simulink model "JenaFox_Klostermair_Neuronal_Controller"  (R2020b)
settings: Solver=ode23s  StartTime=0.0  StopTime=20  MaxStep=maxStep  RelTol=relTol  AbsTol=absTol
InitFcn:
  | Fox_param;
undefined symbols (not defined in the file or in its folder): amplifier, c_coupling_hip, c_coupling_knee, c_hs, d_coupling_knee, d_hs, g, hip_i, hip_Jm, hip_k, hip_Mrg, hip_Mrhg, hip_na, hip_Ra, IC_motor_hip_l, IC_motor_hip_r, IC_motor_knee_l, IC_motor_knee_r, IC_phi_hip_l, IC_phi_hip_r, IC_v_motor_hip, IC_v_motor_knee, k_gx, k_gy, knee_i, knee_Jm, knee_k, knee_Mrg, knee_Mrhg, knee_na, knee_Ra, mu_slide, mu_stick, smiData, v_gx_max, v_gy_max, vLimit, X, Y, Z
libraries: sm_lib x38, nesl_utility x26, simulink x16, simulink_extras x8
(part 2 of 3)

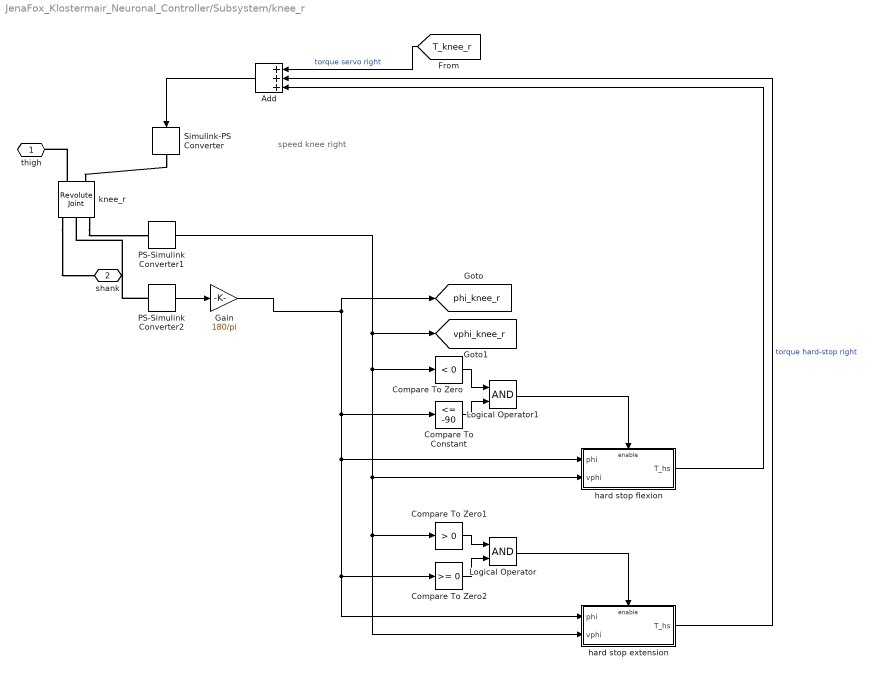
== system JenaFox_Klostermair_Neuronal_Controller/Subsystem/knee_r ==
  note: speed knee right
  Add : Sum  Inputs=+++
  Compare To Constant : simulink/Logic and Bit Operations/Compare To Constant  relop=<=  const=-90  OutDataTypeStr=uint8
  Compare To Zero : simulink/Logic and Bit Operations/Compare To Zero  relop=<  OutDataTypeStr=uint8  ZeroCross=off
  Compare To Zero1 : simulink/Logic and Bit Operations/Compare To Zero  relop=>  OutDataTypeStr=uint8  ZeroCross=off
  Compare To Zero2 : simulink/Logic and Bit Operations/Compare To Zero  relop=>=  OutDataTypeStr=uint8
  Gain : Gain  Gain=180/pi
  Logical Operator : Logic  AllPortsSameDT=off  OutDataTypeStr=boolean
  Logical Operator1 : Logic  AllPortsSameDT=off  OutDataTypeStr=boolean
  PS-Simulink Converter1 : nesl_utility/PS-Simulink Converter  PhysicalDomain=network_engine_domain  SubClassName=ps_output  LeftPortType=input  RightPortType=output  PseudoPeriodic=off  Frequencies=[]  Unit=1  AffineConversion=off
  PS-Simulink Converter2 : nesl_utility/PS-Simulink Converter  PhysicalDomain=network_engine_domain  SubClassName=ps_output  LeftPortType=input  RightPortType=output  PseudoPeriodic=off  Frequencies=[]  Unit=1  AffineConversion=off
  Simulink-PS Converter : nesl_utility/Simulink-PS Converter  PhysicalDomain=network_engine_domain  SubClassName=ps_input  LeftPortType=input  RightPortType=output  PseudoPeriodic=off  Frequencies=[]  NoiseDistribution=none  NoiseParameters=[]  Unit=1  AffineConversion=off  FilteringAndDerivatives=provide  SimscapeFilterOrder=1  InputFilterTimeConstant=0.001  UdotUserProvided=0
  hard stop extension : Subsystem  TreatAsAtomicUnit=on
  hard stop flexion : Subsystem  TreatAsAtomicUnit=on
  knee_r : sm_lib/Joints/Revolute Joint  JointMode=Normal  SenseConstraintForce=off  SenseConstraintForceX=off  SenseConstraintForceY=off  SenseConstraintForceZ=off  SenseConstraintTorque=off  SenseConstraintTorqueX=off  SenseConstraintTorqueY=off  SenseConstraintTorqueZ=off  SenseTotalForce=off  SenseTotalForceX=off  SenseTotalForceY=off  SenseTotalForceZ=off  SenseTotalTorque=off  SenseTotalTorqueX=off  SenseTotalTorqueY=off  SenseTotalTorqueZ=off  CompositeWrenchDir=FollowerOnBase  CompositeWrenchFrame=BaseFrame  EquilibriumPosition=0  EquilibriumPositionUnits=rad  SpringStiffness=0  SpringStiffnessUnits=N*m/rad  DampingCoefficient=d_joint  DampingCoefficientUnits=N*m/(rad/s)  TorqueActuationMode=InputTorque  MotionActuationMode=ComputedMotion  SensePosition=on  SenseVelocity=on  SenseAcceleration=off  SenseTorqueForce=off  SenseLowerLimitTorqueForce=off  SenseUpperLimitTorqueForce=off  LowerLimitSpecify=off  LowerLimitBound=-90  LowerLimitBoundUnits=deg  LowerLimitStiffness=1e4  LowerLimitStiffnessUnits=N*m/deg  LowerLimitDamping=10  LowerLimitDampingUnits=N*m/(deg/s)  LowerLimitTransitionRegionWidth=0.1  LowerLimitTransitionRegionWidthUnits=deg  UpperLimitSpecify=off  UpperLimitBound=90  UpperLimitBoundUnits=deg  UpperLimitStiffness=1e4  UpperLimitStiffnessUnits=N*m/deg  UpperLimitDamping=10  UpperLimitDampingUnits=N*m/(deg/s)  UpperLimitTransitionRegionWidth=0.1  UpperLimitTransitionRegionWidthUnits=deg  PositionTargetSpecify=on  PositionTargetPriority=High  PositionTargetValue=IC_phi_knee_r  PositionTargetValueUnits=deg  VelocityTargetSpecify=off  VelocityTargetPriority=High  VelocityTargetValue=0  VelocityTargetValueUnits=deg/s
  thigh : PMIOPort  Side=Left
  shank : PMIOPort  Port=2  Side=Right
  tag scope: phi_knee_r=global, vphi_knee_r=global
  wires:
  Compare To Constant/1 -> Logical Operator1/2
  PS-Simulink Converter2/1 -> Gain/1
  hard stop extension/1(T_hs) -> Add/2  "torque hard-stop right"
  Compare To Zero1/1 -> Logical Operator/1
  Logical Operator1/1 -> hard stop flexion/Enable
  Logical Operator/1 -> hard stop extension/Enable
  Add/1 -> Simulink-PS Converter/1
  Compare To Zero/1 -> Logical Operator1/1
  PS-Simulink Converter1/1 -> [vphi_knee_r], Compare To Zero/1, hard stop flexion/2(vphi), Compare To Zero1/1, hard stop extension/2(vphi)
  hard stop flexion/1(T_hs) -> Add/3
  Compare To Zero2/1 -> Logical Operator/2
  [T_knee_r] -> Add/1  "torque servo right"
  Gain/1 -> [phi_knee_r], Compare To Constant/1, hard stop flexion/1(phi), Compare To Zero2/1, hard stop extension/1(phi)
  connections:
  Simulink-PS Converter/RConn1 -- knee_r/LConn2
  knee_r/RConn1 -- shank/RConn1
  PS-Simulink Converter2/LConn1 -- knee_r/RConn2
  knee_r/RConn3 -- PS-Simulink Converter1/LConn1
  knee_r/LConn1 -- thigh/RConn1

== system JenaFox_Klostermair_Neuronal_Controller/Subsystem/shank_bottom_l ==
  Rigid Transform : sm_lib/Frames and Transforms/Rigid Transform  TranslationMethod=None  TranslationStandardOffset=0  TranslationLengthUnit=m  TranslationStandardAxis=+Z  TranslationCartesianOffset=[0 0 0]  TranslationROffset=0  TranslationROffsetUnits=m  TranslationZOffset=0  TranslationZOffsetUnits=m  TranslationThetaOffset=0  TranslationThetaOffsetUnits=deg  RotationMethod=AlignedAxes  RotationAngleUnits=deg  RotationStandardAxis=+Z  RotationAngle=0.0  RotationArbitraryAxis=[0 0 1]  FollAlignAxisA=+X  BaseAlignAxisA=-X  FollAlignAxisB=+Z  BaseAlignAxisB=+Y  RotationSequenceAxes=FollowerAxes  RotationSequence=XYX  RotationSequenceAngles=[0 0 0]  RotationSequenceAnglesUnits=deg  RotationMatrix=[1 0 0; 0 1 0; 0 0 1]
  Solid : sm_lib/Body Elements/File Solid  ExtGeomFileName=shank_bottom_ipt_92530788.STEP  UnitType=FromFile  ExtGeomFileUnits=m  StepReaderType=OCC  ExportConvexHullGeometry=off  InertiaType=Custom  Mass=smiData.Solid(4).mass  MassUnits=kg  CenterOfMass=smiData.Solid(4).CoM  CenterOfMassUnits=mm  MomentsOfInertia=smiData.Solid(4).MoI  MomentsOfInertiaUnits=kg*mm^2  ProductsOfInertia=smiData.Solid(4).PoI  ProductsOfInertiaUnits=kg*mm^2  BasedOnType=Density  Density=1000  DensityUnits=kg/m^3  DoExposeReferenceFrame=on  SerializedFrames=<Frames><Frame><Id>Frame1</Id><Value><Name>ground_contact</Name><Origin><Source>GeometricFeature</Source><FeatureName>circular curve 105</FeatureName></Origin><PrimaryAxis><DefinedDirection>+Y</DefinedDirection><Source>ReferenceFrame</Source><SourceDirection>-Y</SourceDirection><FeatureName></FeatureName></PrimaryAxis><SecondaryAxis><DefinedDirection>+X</DefinedDirection><Source>ReferenceFrame</Source><SourceDirection>+X</SourceDirection><FeatureName></FeatureName></SecondaryAxis></Value></Frame><Frame><Id>Frame2</Id><Value><Name>spring_bottom</Name><Origin><Source>GeometricFeature</Source><FeatureName>circular curve 81</FeatureName></Origin><PrimaryAxis><DefinedDirection>+Y</DefinedDirection><Source>ReferenceFrame</Source><SourceDirection>-Y</SourceDirection><FeatureName></FeatureName></PrimaryAxis><SecondaryAxis><DefinedDirection>+X</DefinedDirection><Source>ReferenceFrame</Source><SourceDirection>+X</SourceDirection><FeatureName></FeatureName></SecondaryAxis></Value></Frame></Frames>  GraphicType=FromGeometry  MarkerShape=Sphere  MarkerSize=10  GraphicVisPropType=SimpleVisualProperties  GraphicDiffuseColor=smiData.Solid(4).color  GraphicSpecularColor=[0.5 0.5 0.5 1.0]  GraphicAmbientColor=[0.15 0.15 0.15 1.0]  GraphicEmissiveColor=[0.0 0.0 0.0 1.0]  GraphicShininess=75  GraphicOpacity=smiData.Solid(4).opacity
  linear elastic joint : PMIOPort  Side=Left
  toe : PMIOPort  Port=2  Side=Right
  spring_bottom : PMIOPort  Port=3  Side=Left
  connections:
  toe/RConn1 -- Solid/LConn1
  linear elastic joint/RConn1 -- Rigid Transform/RConn1 -- spring_bottom/RConn1
  Rigid Transform/LConn1 -- Solid/LConn2

== system JenaFox_Klostermair_Neuronal_Controller/Subsystem/shank_bottom_r ==
  Rigid Transform : sm_lib/Frames and Transforms/Rigid Transform  TranslationMethod=None  TranslationStandardOffset=0  TranslationLengthUnit=m  TranslationStandardAxis=+Z  TranslationCartesianOffset=[0 0 0]  TranslationROffset=0  TranslationROffsetUnits=m  TranslationZOffset=0  TranslationZOffsetUnits=m  TranslationThetaOffset=0  TranslationThetaOffsetUnits=deg  RotationMethod=AlignedAxes  RotationAngleUnits=deg  RotationStandardAxis=+Z  RotationAngle=0.0  RotationArbitraryAxis=[0 0 1]  FollAlignAxisA=+X  BaseAlignAxisA=+X  FollAlignAxisB=+Z  BaseAlignAxisB=+Y  RotationSequenceAxes=FollowerAxes  RotationSequence=XYX  RotationSequenceAngles=[0 0 0]  RotationSequenceAnglesUnits=deg  RotationMatrix=[1 0 0; 0 1 0; 0 0 1]
  Solid : sm_lib/Body Elements/File Solid  ExtGeomFileName=shank_bottom_ipt_92530788.STEP  UnitType=FromFile  ExtGeomFileUnits=m  StepReaderType=OCC  ExportConvexHullGeometry=off  InertiaType=Custom  Mass=smiData.Solid(4).mass  MassUnits=kg  CenterOfMass=smiData.Solid(4).CoM  CenterOfMassUnits=mm  MomentsOfInertia=smiData.Solid(4).MoI  MomentsOfInertiaUnits=kg*mm^2  ProductsOfInertia=smiData.Solid(4).PoI  ProductsOfInertiaUnits=kg*mm^2  BasedOnType=Density  Density=1000  DensityUnits=kg/m^3  DoExposeReferenceFrame=off  SerializedFrames=<Frames><Frame><Id>Frame1</Id><Value><Name>ground_contact</Name><Origin><Source>GeometricFeature</Source><FeatureName>circular curve 105</FeatureName></Origin><PrimaryAxis><DefinedDirection>+Y</DefinedDirection><Source>ReferenceFrame</Source><SourceDirection>-Y</SourceDirection><FeatureName></FeatureName></PrimaryAxis><SecondaryAxis><DefinedDirection>+X</DefinedDirection><Source>ReferenceFrame</Source><SourceDirection>+X</SourceDirection><FeatureName></FeatureName></SecondaryAxis></Value></Frame><Frame><Id>Frame2</Id><Value><Name>spring_bottom</Name><Origin><Source>GeometricFeature</Source><FeatureName>circular curve 81</FeatureName></Origin><PrimaryAxis><DefinedDirection>+Y</DefinedDirection><Source>ReferenceFrame</Source><SourceDirection>-Y</SourceDirection><FeatureName></FeatureName></PrimaryAxis><SecondaryAxis><DefinedDirection>+X</DefinedDirection><Source>ReferenceFrame</Source><SourceDirection>+X</SourceDirection><FeatureName></FeatureName></SecondaryAxis></Value></Frame></Frames>  GraphicType=FromGeometry  MarkerShape=Sphere  MarkerSize=10  GraphicVisPropType=SimpleVisualProperties  GraphicDiffuseColor=smiData.Solid(4).color  GraphicSpecularColor=[0.5 0.5 0.5 1.0]  GraphicAmbientColor=[0.15 0.15 0.15 1.0]  GraphicEmissiveColor=[0.0 0.0 0.0 1.0]  GraphicShininess=75  GraphicOpacity=smiData.Solid(4).opacity
  linear elastic joint : PMIOPort  Side=Left
  toe : PMIOPort  Port=2  Side=Right
  spring_bottom : PMIOPort  Port=3  Side=Left
  connections:
  toe/RConn1 -- Solid/LConn1
  linear elastic joint/RConn1 -- Rigid Transform/RConn1 -- spring_bottom/RConn1
  Rigid Transform/LConn1 -- Solid/RConn1

== system JenaFox_Klostermair_Neuronal_Controller/Subsystem/shank_top_l ==
  Rigid Transform : sm_lib/Frames and Transforms/Rigid Transform  TranslationMethod=StandardAxis  TranslationStandardOffset=0.11  TranslationLengthUnit=m  TranslationStandardAxis=+Z  TranslationCartesianOffset=[0 0 0]  TranslationROffset=0  TranslationROffsetUnits=m  TranslationZOffset=0  TranslationZOffsetUnits=m  TranslationThetaOffset=0  TranslationThetaOffsetUnits=deg  RotationMethod=AlignedAxes  RotationAngleUnits=deg  RotationStandardAxis=+Z  RotationAngle=0.0  RotationArbitraryAxis=[0 0 1]  FollAlignAxisA=+X  BaseAlignAxisA=+X  FollAlignAxisB=+Y  BaseAlignAxisB=+Z  RotationSequenceAxes=FollowerAxes  RotationSequence=XYX  RotationSequenceAngles=[0 0 0]  RotationSequenceAnglesUnits=deg  RotationMatrix=[1 0 0; 0 1 0; 0 0 1]
  Solid : sm_lib/Body Elements/File Solid  ExtGeomFileName=shank_top_ipt_5be12039.STEP  UnitType=FromFile  ExtGeomFileUnits=m  StepReaderType=OCC  ExportConvexHullGeometry=off  InertiaType=Custom  Mass=smiData.Solid(3).mass  MassUnits=kg  CenterOfMass=smiData.Solid(3).CoM  CenterOfMassUnits=mm  MomentsOfInertia=smiData.Solid(3).MoI  MomentsOfInertiaUnits=kg*mm^2  ProductsOfInertia=smiData.Solid(3).PoI  ProductsOfInertiaUnits=kg*mm^2  BasedOnType=Density  Density=1000  DensityUnits=kg/m^3  DoExposeReferenceFrame=off  SerializedFrames=<Frames><Frame><Id>Frame1</Id><Value><Name>spring_top</Name><Origin><Source>GeometricFeature</Source><FeatureName>circular curve 166</FeatureName></Origin><PrimaryAxis><DefinedDirection>+Y</DefinedDirection><Source>ReferenceFrame</Source><SourceDirection>-Y</SourceDirection><FeatureName></FeatureName></PrimaryAxis><SecondaryAxis><DefinedDirection>+X</DefinedDirection><Source>GeometricFeature</Source><SourceDirection>+X</SourceDirection><FeatureName>segment 110</FeatureName></SecondaryAxis></Value></Frame><Frame><Id>Frame2</Id><Value><Name>knee</Name><Origin><Source>GeometricFeature</Source><FeatureName>circular curve 135</FeatureName></Origin><PrimaryAxis><DefinedDirection>-X</DefinedDirection><Source>GeometricFeature</Source><SourceDirection>+Z</SourceDirection><FeatureName>segment 80</FeatureName></PrimaryAxis><SecondaryAxis><DefinedDirection>+Y</DefinedDirection><Source>GeometricFeature</Source><SourceDirection>+X</SourceDirection><FeatureName>segment 115</FeatureName></SecondaryAxis></Value></Frame></Frames>  GraphicType=FromGeometry  MarkerShape=Sphere  MarkerSize=10  GraphicVisPropType=SimpleVisualProperties  GraphicDiffuseColor=smiData.Solid(3).color  GraphicSpecularColor=[0.5 0.5 0.5 1.0]  GraphicAmbientColor=[0.15 0.15 0.15 1.0]  GraphicEmissiveColor=[0.0 0.0 0.0 1.0]  GraphicShininess=75  GraphicOpacity=smiData.Solid(3).opacity
  knee : PMIOPort  Side=Left
  linear joint : PMIOPort  Port=2  Side=Right
  spring_top : PMIOPort  Port=3  Side=Right
  connections:
  knee/RConn1 -- Solid/RConn1
  Rigid Transform/RConn1 -- spring_top/RConn1 -- Solid/LConn1
  linear joint/RConn1 -- Rigid Transform/LConn1

== system JenaFox_Klostermair_Neuronal_Controller/Subsystem/shank_top_r ==
  Rigid Transform : sm_lib/Frames and Transforms/Rigid Transform  TranslationMethod=StandardAxis  TranslationStandardOffset=0.11  TranslationLengthUnit=m  TranslationStandardAxis=+Z  TranslationCartesianOffset=[0 0 0]  TranslationROffset=0  TranslationROffsetUnits=m  TranslationZOffset=0  TranslationZOffsetUnits=m  TranslationThetaOffset=0  TranslationThetaOffsetUnits=deg  RotationMethod=AlignedAxes  RotationAngleUnits=deg  RotationStandardAxis=+Z  RotationAngle=0.0  RotationArbitraryAxis=[0 0 1]  FollAlignAxisA=+X  BaseAlignAxisA=+X  FollAlignAxisB=+Y  BaseAlignAxisB=+Z  RotationSequenceAxes=FollowerAxes  RotationSequence=XYX  RotationSequenceAngles=[0 0 0]  RotationSequenceAnglesUnits=deg  RotationMatrix=[1 0 0; 0 1 0; 0 0 1]
  Solid : sm_lib/Body Elements/File Solid  ExtGeomFileName=shank_top_ipt_5be12039.STEP  UnitType=FromFile  ExtGeomFileUnits=m  StepReaderType=OCC  ExportConvexHullGeometry=off  InertiaType=Custom  Mass=smiData.Solid(3).mass  MassUnits=kg  CenterOfMass=smiData.Solid(3).CoM  CenterOfMassUnits=mm  MomentsOfInertia=smiData.Solid(3).MoI  MomentsOfInertiaUnits=kg*mm^2  ProductsOfInertia=smiData.Solid(3).PoI  ProductsOfInertiaUnits=kg*mm^2  BasedOnType=Density  Density=1000  DensityUnits=kg/m^3  DoExposeReferenceFrame=off  SerializedFrames=<Frames><Frame><Id>Frame1</Id><Value><Name>spring_top</Name><Origin><Source>GeometricFeature</Source><FeatureName>circular curve 166</FeatureName></Origin><PrimaryAxis><DefinedDirection>+Y</DefinedDirection><Source>ReferenceFrame</Source><SourceDirection>-Y</SourceDirection><FeatureName></FeatureName></PrimaryAxis><SecondaryAxis><DefinedDirection>+X</DefinedDirection><Source>GeometricFeature</Source><SourceDirection>+X</SourceDirection><FeatureName>segment 110</FeatureName></SecondaryAxis></Value></Frame><Frame><Id>Frame2</Id><Value><Name>shank_knee_right</Name><Origin><Source>GeometricFeature</Source><FeatureName>circular curve 135</FeatureName></Origin><PrimaryAxis><DefinedDirection>+X</DefinedDirection><Source>GeometricFeature</Source><SourceDirection>+Z</SourceDirection><FeatureName>segment 110</FeatureName></PrimaryAxis><SecondaryAxis><DefinedDirection>+Y</DefinedDirection><Source>GeometricFeature</Source><SourceDirection>+X</SourceDirection><FeatureName>segment 138</FeatureName></SecondaryAxis></Value></Frame></Frames>  GraphicType=FromGeometry  MarkerShape=Sphere  MarkerSize=10  GraphicVisPropType=SimpleVisualProperties  GraphicDiffuseColor=smiData.Solid(3).color  GraphicSpecularColor=[0.5 0.5 0.5 1.0]  GraphicAmbientColor=[0.15 0.15 0.15 1.0]  GraphicEmissiveColor=[0.0 0.0 0.0 1.0]  GraphicShininess=75  GraphicOpacity=smiData.Solid(3).opacity
  knee : PMIOPort  Side=Left
  linear joint : PMIOPort  Port=2  Side=Right
  spring_top : PMIOPort  Port=3  Side=Right
  connections:
  knee/RConn1 -- Solid/RConn1
  Rigid Transform/RConn1 -- spring_top/RConn1 -- Solid/LConn1
  linear joint/RConn1 -- Rigid Transform/LConn1

== system JenaFox_Klostermair_Neuronal_Controller/Subsystem/thigh_l ==
  Solid : sm_lib/Body Elements/File Solid  ExtGeomFileName=thigh_left_ipt_d01cdd9b.STEP  UnitType=FromFile  ExtGeomFileUnits=m  StepReaderType=OCC  ExportConvexHullGeometry=off  InertiaType=Custom  Mass=smiData.Solid(2).mass  MassUnits=kg  CenterOfMass=smiData.Solid(2).CoM  CenterOfMassUnits=mm  MomentsOfInertia=smiData.Solid(2).MoI  MomentsOfInertiaUnits=kg*mm^2  ProductsOfInertia=smiData.Solid(2).PoI  ProductsOfInertiaUnits=kg*mm^2  BasedOnType=Density  Density=1000  DensityUnits=kg/m^3  DoExposeReferenceFrame=off  SerializedFrames=<Frames><Frame><Id>Frame1</Id><Value><Name>thigh_left_knee</Name><Origin><Source>GeometricFeature</Source><FeatureName>planar surface 172</FeatureName></Origin><PrimaryAxis><DefinedDirection>+Z</DefinedDirection><Source>ReferenceFrame</Source><SourceDirection>-Y</SourceDirection><FeatureName></FeatureName></PrimaryAxis><SecondaryAxis><DefinedDirection>+X</DefinedDirection><Source>ReferenceFrame</Source><SourceDirection>+X</SourceDirection><FeatureName></FeatureName></SecondaryAxis></Value></Frame><Frame><Id>Frame2</Id><Value><Name>thigh_left_hip</Name><Origin><Source>GeometricFeature</Source><FeatureName>circular curve 156</FeatureName></Origin><PrimaryAxis><DefinedDirection>+Z</DefinedDirection><Source>ReferenceFrame</Source><SourceDirection>-Y</SourceDirection><FeatureName></FeatureName></PrimaryAxis><SecondaryAxis><DefinedDirection>+X</DefinedDirection><Source>ReferenceFrame</Source><SourceDirection>+X</SourceDirection><FeatureName></FeatureName></SecondaryAxis></Value></Frame></Frames>  GraphicType=FromGeometry  MarkerShape=Sphere  MarkerSize=10  GraphicVisPropType=SimpleVisualProperties  GraphicDiffuseColor=smiData.Solid(2).color  GraphicSpecularColor=[0.5 0.5 0.5 1.0]  GraphicAmbientColor=[0.15 0.15 0.15 1.0]  GraphicEmissiveColor=[0.0 0.0 0.0 1.0]  GraphicShininess=75  GraphicOpacity=smiData.Solid(2).opacity
  hip : PMIOPort  Side=Left
  knee : PMIOPort  Port=2  Side=Right
  connections:
  hip/RConn1 -- Solid/RConn1
  knee/RConn1 -- Solid/LConn1

== system JenaFox_Klostermair_Neuronal_Controller/Subsystem/thigh_r ==
  Solid : sm_lib/Body Elements/File Solid  ExtGeomFileName=thigh_left_ipt_d01cdd9b.STEP  UnitType=FromFile  ExtGeomFileUnits=m  StepReaderType=OCC  ExportConvexHullGeometry=off  InertiaType=Custom  Mass=smiData.Solid(2).mass  MassUnits=kg  CenterOfMass=smiData.Solid(2).CoM  CenterOfMassUnits=mm  MomentsOfInertia=smiData.Solid(2).MoI  MomentsOfInertiaUnits=kg*mm^2  ProductsOfInertia=smiData.Solid(2).PoI  ProductsOfInertiaUnits=kg*mm^2  BasedOnType=Density  Density=1000  DensityUnits=kg/m^3  DoExposeReferenceFrame=off  SerializedFrames=<Frames><Frame><Id>Frame1</Id><Value><Name>thigh_right_knee</Name><Origin><Source>GeometricFeature</Source><FeatureName>circular curve 616</FeatureName></Origin><PrimaryAxis><DefinedDirection>+Z</DefinedDirection><Source>ReferenceFrame</Source><SourceDirection>+Y</SourceDirection><FeatureName></FeatureName></PrimaryAxis><SecondaryAxis><DefinedDirection>+X</DefinedDirection><Source>ReferenceFrame</Source><SourceDirection>-X</SourceDirection><FeatureName></FeatureName></SecondaryAxis></Value></Frame><Frame><Id>Frame2</Id><Value><Name>thigh_right_hip</Name><Origin><Source>GeometricFeature</Source><FeatureName>circular curve 280</FeatureName></Origin><PrimaryAxis><DefinedDirection>+Z</DefinedDirection><Source>ReferenceFrame</Source><SourceDirection>+Y</SourceDirection><FeatureName></FeatureName></PrimaryAxis><SecondaryAxis><DefinedDirection>+X</DefinedDirection><Source>ReferenceFrame</Source><SourceDirection>-X</SourceDirection><FeatureName></FeatureName></SecondaryAxis></Value></Frame></Frames>  GraphicType=FromGeometry  MarkerShape=Sphere  MarkerSize=10  GraphicVisPropType=SimpleVisualProperties  GraphicDiffuseColor=smiData.Solid(2).color  GraphicSpecularColor=[0.5 0.5 0.5 1.0]  GraphicAmbientColor=[0.15 0.15 0.15 1.0]  GraphicEmissiveColor=[0.0 0.0 0.0 1.0]  GraphicShininess=75  GraphicOpacity=smiData.Solid(2).opacity
  hip : PMIOPort  Side=Left
  knee : PMIOPort  Port=2  Side=Right
  connections:
  knee/RConn1 -- Solid/LConn1
  Solid/RConn1 -- hip/RConn1

== system JenaFox_Klostermair_Neuronal_Controller/Subsystem/trunk ==
  Solid : sm_lib/Body Elements/File Solid  ExtGeomFileName=trunk_ipt_7785b5f2.STEP  UnitType=FromFile  ExtGeomFileUnits=m  StepReaderType=OCC  ExportConvexHullGeometry=off  InertiaType=Custom  Mass=smiData.Solid(1).mass  MassUnits=kg  CenterOfMass=smiData.Solid(1).CoM  CenterOfMassUnits=mm  MomentsOfInertia=smiData.Solid(1).MoI  MomentsOfInertiaUnits=kg*mm^2  ProductsOfInertia=smiData.Solid(1).PoI  ProductsOfInertiaUnits=kg*mm^2  BasedOnType=Density  Density=1000  DensityUnits=kg/m^3  DoExposeReferenceFrame=off  SerializedFrames=<Frames><Frame><Id>Frame1</Id><Value><Name>hip_right</Name><Origin><Source>GeometricFeature</Source><FeatureName>circular curve 591</FeatureName></Origin><PrimaryAxis><DefinedDirection>+Z</DefinedDirection><Source>ReferenceFrame</Source><SourceDirection>+X</SourceDirection><FeatureName></FeatureName></PrimaryAxis><SecondaryAxis><DefinedDirection>+X</DefinedDirection><Source>ReferenceFrame</Source><SourceDirection>-Z</SourceDirection><FeatureName></FeatureName></SecondaryAxis></Value></Frame><Frame><Id>Frame2</Id><Value><Name>hip_left</Name><Origin><Source>GeometricFeature</Source><FeatureName>circular curve 612</FeatureName></Origin><PrimaryAxis><DefinedDirection>+Z</DefinedDirection><Source>ReferenceFrame</Source><SourceDirection>+X</SourceDirection><FeatureName></FeatureName></PrimaryAxis><SecondaryAxis><DefinedDirection>+X</DefinedDirection><Source>ReferenceFrame</Source><SourceDirection>-Z</SourceDirection><FeatureName></FeatureName></SecondaryAxis></Value></Frame><Frame><Id>Frame3</Id><Value><Name>boom_connector</Name><Origin><Source>GeometricFeature</Source><FeatureName>circular curve 1475</FeatureName></Origin><PrimaryAxis><DefinedDirection>+X</DefinedDirection><Source>ReferenceFrame</Source><SourceDirection>-Z</SourceDirection><FeatureName></FeatureName></PrimaryAxis><SecondaryAxis><DefinedDirection>+Y</DefinedDirection><Source>ReferenceFrame</Source><SourceDirection>+Y</SourceDirection><FeatureName></FeatureName></SecondaryAxis></Value></Frame></Frames>  GraphicType=FromGeometry  MarkerShape=Sphere  MarkerSize=10  GraphicVisPropType=SimpleVisualProperties  GraphicDiffuseColor=smiData.Solid(1).color  GraphicSpecularColor=[0.5 0.5 0.5 1.0]  GraphicAmbientColor=[0.15 0.15 0.15 1.0]  GraphicEmissiveColor=[0.0 0.0 0.0 1.0]  GraphicShininess=75  GraphicOpacity=smiData.Solid(1).opacity
  hip left : PMIOPort  Side=Right
  hip right : PMIOPort  Port=2  Side=Right
  boom : PMIOPort  Port=3  Side=Left
  connections:
  Solid/RConn1 -- hip left/RConn1
  hip right/RConn1 -- Solid/LConn1
  boom/RConn1 -- Solid/LConn2

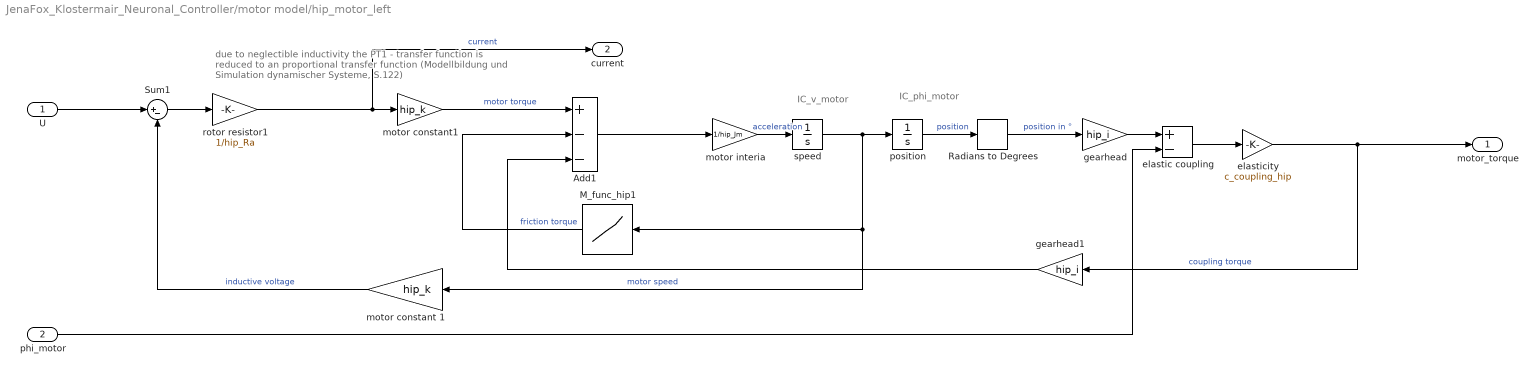
== system JenaFox_Klostermair_Neuronal_Controller/motor model/hip_motor_left ==
  note: IC_phi_motor
  note: IC_v_motor
  note: due to neglectible inductivity the
      | PT1 - transfer function is reduced to an
      | proportional transfer function
      | (Modellbildung und Simulation dynamischer Systeme, S.122)
  U : Inport
  phi_motor : Inport  Port=2
  Add1 : Sum  Inputs=+--
  M_func_hip1 : Lookup  InputValues=[-10^10 -hip_na -0.001 0 0.001 hip_na 10^10]  Table=[-hip_Mrg -hip_Mrg -hip_Mrhg 0 hip_Mrhg hip_Mrg hip_Mrg]
  Radians to Degrees : simulink_extras/Transformations/Radians to Degrees
  Sum1 : Sum  Inputs=|+-
  elastic coupling : Sum  Inputs=+-
  elasticity : Gain  Gain=c_coupling_hip
  gearhead : Gain  Gain=hip_i
  gearhead1 : Gain  Gain=hip_i
  motor constant 1 : Gain  Gain=hip_k
  motor constant1 : Gain  Gain=hip_k
  motor interia : Gain  Gain=1/hip_Jm
  position : Integrator  InitialCondition=IC_motor_hip_l  ContinuousStateAttributes='position_hip'
  rotor resistor1 : Gain  Gain=1/hip_Ra
  speed : Integrator  InitialCondition=IC_v_motor_hip  ContinuousStateAttributes='speed_hip'
  motor_torque : Outport  VectorParamsAs1DForOutWhenUnconnected=off
  current : Outport  Port=2  VectorParamsAs1DForOutWhenUnconnected=off
  wires:
  elasticity/1 -> motor_torque/1, gearhead1/1  "coupling torque"
  gearhead1/1 -> Add1/3
  phi_motor/1 -> elastic coupling/2
  U/1 -> Sum1/1
  Radians to Degrees/1 -> gearhead/1  "position in °"
  gearhead/1 -> elastic coupling/1
  elastic coupling/1 -> elasticity/1
  position/1 -> Radians to Degrees/1  "position"
  motor constant 1/1 -> Sum1/2  "inductive voltage"
  speed/1 -> motor constant 1/1, M_func_hip1/1, position/1  "motor speed"
  Sum1/1 -> rotor resistor1/1
  motor interia/1 -> speed/1  "acceleration"
  Add1/1 -> motor interia/1
  M_func_hip1/1 -> Add1/2  "friction torque"
  motor constant1/1 -> Add1/1  "motor torque"
  rotor resistor1/1 -> current/1, motor constant1/1  "current"

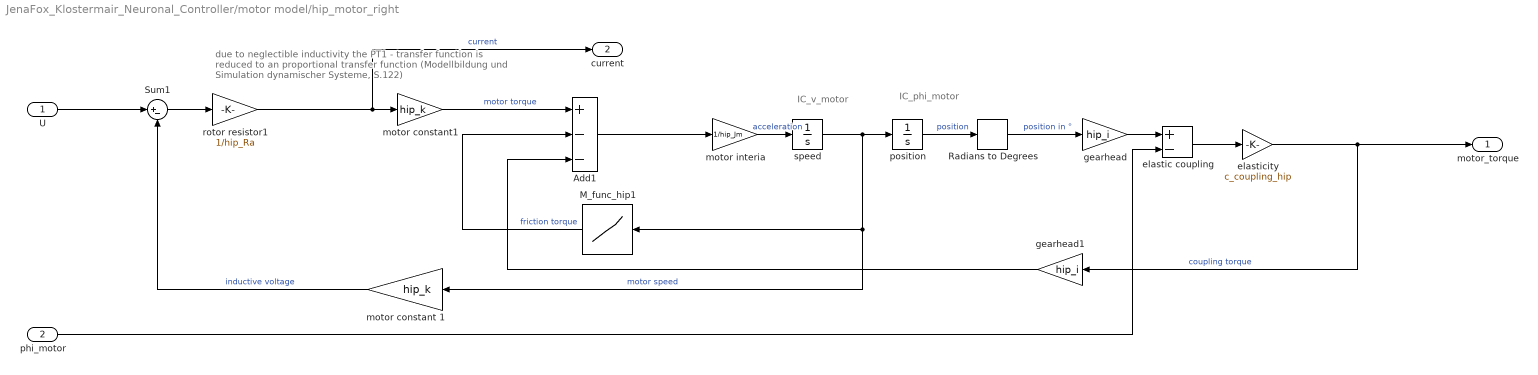
== system JenaFox_Klostermair_Neuronal_Controller/motor model/hip_motor_right ==
  note: IC_phi_motor
  note: IC_v_motor
  note: due to neglectible inductivity the
      | PT1 - transfer function is reduced to an
      | proportional transfer function
      | (Modellbildung und Simulation dynamischer Systeme, S.122)
  U : Inport
  phi_motor : Inport  Port=2
  Add1 : Sum  Inputs=+--
  M_func_hip1 : Lookup  InputValues=[-10^10 -hip_na -0.001 0 0.001 hip_na 10^10]  Table=[-hip_Mrg -hip_Mrg -hip_Mrhg 0 hip_Mrhg hip_Mrg hip_Mrg]
  Radians to Degrees : simulink_extras/Transformations/Radians to Degrees
  Sum1 : Sum  Inputs=|+-
  elastic coupling : Sum  Inputs=+-
  elasticity : Gain  Gain=c_coupling_hip
  gearhead : Gain  Gain=hip_i
  gearhead1 : Gain  Gain=hip_i
  motor constant 1 : Gain  Gain=hip_k
  motor constant1 : Gain  Gain=hip_k
  motor interia : Gain  Gain=1/hip_Jm
  position : Integrator  InitialCondition=IC_motor_hip_r  ContinuousStateAttributes='position_hip'
  rotor resistor1 : Gain  Gain=1/hip_Ra
  speed : Integrator  InitialCondition=IC_v_motor_hip  ContinuousStateAttributes='speed_hip'
  motor_torque : Outport  VectorParamsAs1DForOutWhenUnconnected=off
  current : Outport  Port=2  VectorParamsAs1DForOutWhenUnconnected=off
  wires:
  elasticity/1 -> motor_torque/1, gearhead1/1  "coupling torque"
  gearhead1/1 -> Add1/3
  phi_motor/1 -> elastic coupling/2
  U/1 -> Sum1/1
  Radians to Degrees/1 -> gearhead/1  "position in °"
  gearhead/1 -> elastic coupling/1
  elastic coupling/1 -> elasticity/1
  position/1 -> Radians to Degrees/1  "position"
  motor constant 1/1 -> Sum1/2  "inductive voltage"
  speed/1 -> motor constant 1/1, M_func_hip1/1, position/1  "motor speed"
  Sum1/1 -> rotor resistor1/1
  motor interia/1 -> speed/1  "acceleration"
  Add1/1 -> motor interia/1
  M_func_hip1/1 -> Add1/2  "friction torque"
  motor constant1/1 -> Add1/1  "motor torque"
  rotor resistor1/1 -> current/1, motor constant1/1  "current"

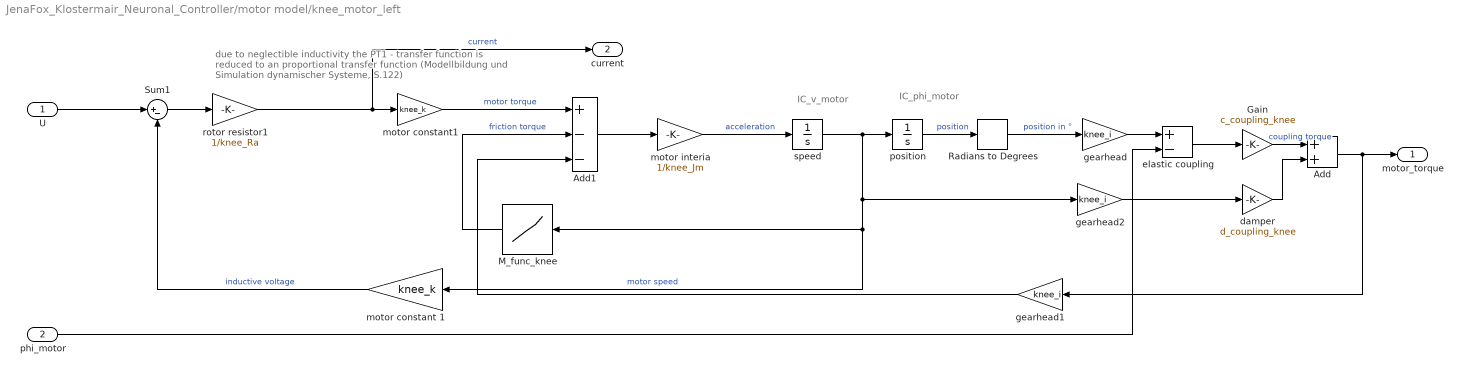
== system JenaFox_Klostermair_Neuronal_Controller/motor model/knee_motor_left ==
  note: due to neglectible inductivity the
      | PT1 - transfer function is reduced to an
      | proportional transfer function
      | (Modellbildung und Simulation dynamischer Systeme, S.122)
  note: IC_v_motor
  note: IC_phi_motor
  U : Inport
  phi_motor : Inport  Port=2
  Add : Sum
  Add1 : Sum  Inputs=+--
  Gain : Gain  Gain=c_coupling_knee
  M_func_knee : Lookup  InputValues=[-10^10 -knee_na -0.001 0 0.001 knee_na 10^10]  Table=[-knee_Mrg -knee_Mrg -knee_Mrhg 0 knee_Mrhg knee_Mrg knee_Mrg]
  Radians to Degrees : simulink_extras/Transformations/Radians to Degrees
  Sum1 : Sum  Inputs=|+-
  damper : Gain  Gain=d_coupling_knee
  elastic coupling : Sum  Inputs=+-
  gearhead : Gain  Gain=knee_i
  gearhead1 : Gain  Gain=knee_i
  gearhead2 : Gain  Gain=knee_i
  motor constant 1 : Gain  Gain=knee_k
  motor constant1 : Gain  Gain=knee_k
  motor interia : Gain  Gain=1/knee_Jm
  position : Integrator  InitialCondition=IC_motor_knee_l  ContinuousStateAttributes='position_hip'
  rotor resistor1 : Gain  Gain=1/knee_Ra
  speed : Integrator  InitialCondition=IC_v_motor_knee  ContinuousStateAttributes='speed_hip'
  motor_torque : Outport  VectorParamsAs1DForOutWhenUnconnected=off
  current : Outport  Port=2  VectorParamsAs1DForOutWhenUnconnected=off
  wires:
  gearhead1/1 -> Add1/3
  rotor resistor1/1 -> motor constant1/1, current/1  "current"
  motor constant1/1 -> Add1/1  "motor torque"
  M_func_knee/1 -> Add1/2  "friction torque"
  Add1/1 -> motor interia/1
  motor interia/1 -> speed/1  "acceleration"
  Sum1/1 -> rotor resistor1/1
  speed/1 -> position/1, M_func_knee/1, motor constant 1/1, gearhead2/1  "motor speed"
  position/1 -> Radians to Degrees/1  "position"
  elastic coupling/1 -> Gain/1
  gearhead/1 -> elastic coupling/1
  Radians to Degrees/1 -> gearhead/1  "position in °"
  U/1 -> Sum1/1
  phi_motor/1 -> elastic coupling/2
  motor constant 1/1 -> Sum1/2  "inductive voltage"
  Gain/1 -> Add/1  "coupling torque"
  Add/1 -> motor_torque/1, gearhead1/1
  gearhead2/1 -> damper/1
  damper/1 -> Add/2

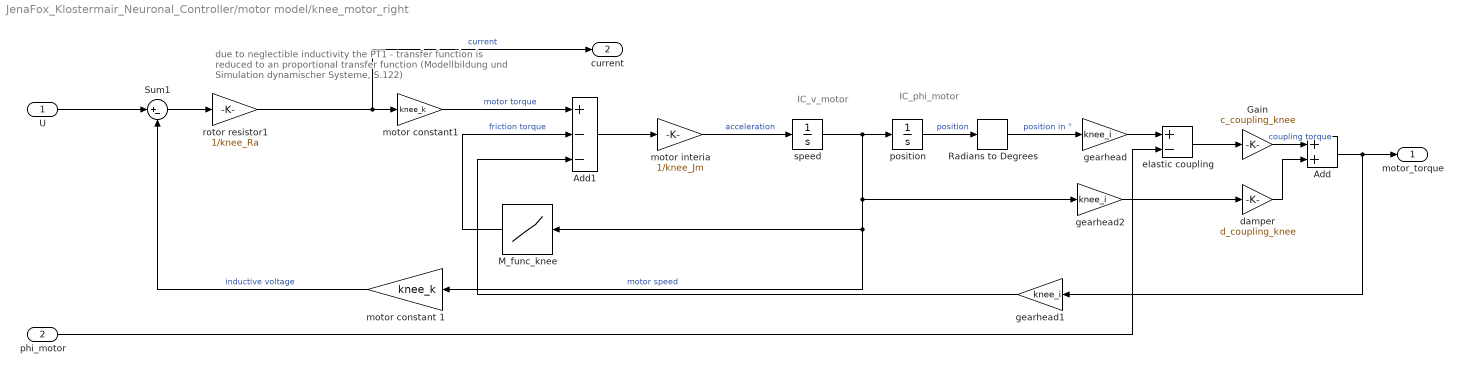
== system JenaFox_Klostermair_Neuronal_Controller/motor model/knee_motor_right ==
  note: due to neglectible inductivity the
      | PT1 - transfer function is reduced to an
      | proportional transfer function
      | (Modellbildung und Simulation dynamischer Systeme, S.122)
  note: IC_v_motor
  note: IC_phi_motor
  U : Inport
  phi_motor : Inport  Port=2
  Add : Sum
  Add1 : Sum  Inputs=+--
  Gain : Gain  Gain=c_coupling_knee
  M_func_knee : Lookup  InputValues=[-10^10 -knee_na -0.001 0 0.001 knee_na 10^10]  Table=[-knee_Mrg -knee_Mrg -knee_Mrhg 0 knee_Mrhg knee_Mrg knee_Mrg]
  Radians to Degrees : simulink_extras/Transformations/Radians to Degrees
  Sum1 : Sum  Inputs=|+-
  damper : Gain  Gain=d_coupling_knee
  elastic coupling : Sum  Inputs=+-
  gearhead : Gain  Gain=knee_i
  gearhead1 : Gain  Gain=knee_i
  gearhead2 : Gain  Gain=knee_i
  motor constant 1 : Gain  Gain=knee_k
  motor constant1 : Gain  Gain=knee_k
  motor interia : Gain  Gain=1/knee_Jm
  position : Integrator  InitialCondition=IC_phi_motor_knee  ContinuousStateAttributes='position_hip'
  rotor resistor1 : Gain  Gain=1/knee_Ra
  speed : Integrator  InitialCondition=IC_v_motor_knee  ContinuousStateAttributes='speed_hip'
  motor_torque : Outport  VectorParamsAs1DForOutWhenUnconnected=off
  current : Outport  Port=2  VectorParamsAs1DForOutWhenUnconnected=off
  wires:
  gearhead1/1 -> Add1/3
  rotor resistor1/1 -> motor constant1/1, current/1  "current"
  motor constant1/1 -> Add1/1  "motor torque"
  M_func_knee/1 -> Add1/2  "friction torque"
  Add1/1 -> motor interia/1
  motor interia/1 -> speed/1  "acceleration"
  Sum1/1 -> rotor resistor1/1
  speed/1 -> position/1, M_func_knee/1, motor constant 1/1, gearhead2/1  "motor speed"
  position/1 -> Radians to Degrees/1  "position"
  elastic coupling/1 -> Gain/1
  gearhead/1 -> elastic coupling/1
  Radians to Degrees/1 -> gearhead/1  "position in °"
  U/1 -> Sum1/1
  phi_motor/1 -> elastic coupling/2
  motor constant 1/1 -> Sum1/2  "inductive voltage"
  Gain/1 -> Add/1  "coupling torque"
  Add/1 -> motor_torque/1, gearhead1/1
  gearhead2/1 -> damper/1
  damper/1 -> Add/2

== system JenaFox_Klostermair_Neuronal_Controller/Subsystem/Ground Contact Model/Ground Friction Model ==
  note: Horizontal Ground Friction Model
  note: Vertical Ground Stiction Model
  dy [m] : Inport
  vy [m/s] : Inport  Port=2
  x [m] : Inport  Port=3
  vx [m/s] : Inport  Port=4
  Contact! : EnablePort  StatesWhenEnabling=reset  PropagateVarSize=During execution
  Data Type Conversion : DataTypeConversion  OutDataTypeStr=double
  Friction Switch : Subsystem
  Gain3 : Gain  Gain=k_gy
  Gain4 : Gain  Gain=1/v_gy_max
  Logical Operator : Logic  Operator=NOT  AllPortsSameDT=off  OutDataTypeStr=boolean
  Mux1 : Mux  Inputs=2
  Sum1 : Sum
  X-Axis Kinetic Friction Model : Subsystem
  X-Axis Static Friction Model : Subsystem
  Y-Axis Ground Force : Fcn  Expr="- u(1)  *  (1-u(2)) * (u(2)<1)"
  Fy_Ground[N] : Outport  OutputWhenDisabled=reset  InitialOutput=0  VectorParamsAs1DForOutWhenUnconnected=off
      settings: AttributesFormatString=initial = '%<InitialOutput>'\nwhen disabled = '%<OutputWhenDisabled>'
  Fx_Friction [N] : Outport  Port=2  OutputWhenDisabled=reset  InitialOutput=0  VectorParamsAs1DForOutWhenUnconnected=off
      settings: AttributesFormatString=initial = '%<InitialOutput>'\nwhen\ndisabled\n'%<OutputWhenDisabled>'
  Stiction! : Outport  Port=3  OutputWhenDisabled=reset  InitialOutput=0  VectorParamsAs1DForOutWhenUnconnected=off
      settings: AttributesFormatString=initial = '%<InitialOutput>'\nwhen\ndisabled\n'%<OutputWhenDisabled>'
  wires:
  dy [m]/1 -> Gain3/1
  vy [m/s]/1 -> Gain4/1
  x [m]/1 -> X-Axis Static Friction Model/2(pos [m]), X-Axis Kinetic Friction Model/1(pos [m])
  vx [m/s]/1 -> X-Axis Static Friction Model/3(vel [m/s]), X-Axis Kinetic Friction Model/2(vel [m/s])
  X-Axis Kinetic Friction Model/1(posFP [m]) -> X-Axis Static Friction Model/4(posFP [m])
  X-Axis Kinetic Friction Model/3(F_Slide [N]) -> Sum1/2
  X-Axis Static Friction Model/1(F_Stick [N]) -> Sum1/1
  Sum1/1 -> Fx_Friction [N]/1
  Friction Switch/1(Stiction) -> X-Axis Static Friction Model/Enable, Logical Operator/1, Data Type Conversion/1
  X-Axis Static Friction Model/2(Sliding!) -> Friction Switch/1(Slide!)
  X-Axis Kinetic Friction Model/2(Stiction!) -> Friction Switch/2(Stick!)
  Logical Operator/1 -> X-Axis Kinetic Friction Model/Enable
  Data Type Conversion/1 -> Stiction!/1
  Mux1/1 -> Y-Axis Ground Force/1
  Gain3/1 -> Mux1/1
  Gain4/1 -> Mux1/2
  Y-Axis Ground Force/1 -> Fy_Ground[N]/1, X-Axis Static Friction Model/1(F_Normal [N]), X-Axis Kinetic Friction Model/3(F_Normal [N])

== system JenaFox_Klostermair_Neuronal_Controller/Subsystem/Ground Contact Model1/Ground Friction Model ==
  note: Horizontal Ground Friction Model
  note: Vertical Ground Stiction Model
  dy [m] : Inport
  vy [m/s] : Inport  Port=2
  x [m] : Inport  Port=3
  vx [m/s] : Inport  Port=4
  Contact! : EnablePort  StatesWhenEnabling=reset  PropagateVarSize=During execution
  Data Type Conversion : DataTypeConversion  OutDataTypeStr=double
  Friction Switch : Subsystem
  Gain3 : Gain  Gain=k_gy
  Gain4 : Gain  Gain=1/v_gy_max
  Logical Operator : Logic  Operator=NOT  AllPortsSameDT=off  OutDataTypeStr=boolean
  Mux1 : Mux  Inputs=2
  Sum1 : Sum
  X-Axis Kinetic Friction Model : Subsystem
  X-Axis Static Friction Model : Subsystem
  Y-Axis Ground Force : Fcn  Expr="- u(1)  *  (1-u(2)) * (u(2)<1)"
  Fy_Ground[N] : Outport  OutputWhenDisabled=reset  InitialOutput=0  VectorParamsAs1DForOutWhenUnconnected=off
      settings: AttributesFormatString=initial = '%<InitialOutput>'\nwhen disabled = '%<OutputWhenDisabled>'
  Fx_Friction [N] : Outport  Port=2  OutputWhenDisabled=reset  InitialOutput=0  VectorParamsAs1DForOutWhenUnconnected=off
      settings: AttributesFormatString=initial = '%<InitialOutput>'\nwhen\ndisabled\n'%<OutputWhenDisabled>'
  Stiction! : Outport  Port=3  OutputWhenDisabled=reset  InitialOutput=0  VectorParamsAs1DForOutWhenUnconnected=off
      settings: AttributesFormatString=initial = '%<InitialOutput>'\nwhen\ndisabled\n'%<OutputWhenDisabled>'
  wires:
  dy [m]/1 -> Gain3/1
  vy [m/s]/1 -> Gain4/1
  x [m]/1 -> X-Axis Static Friction Model/2(pos [m]), X-Axis Kinetic Friction Model/1(pos [m])
  vx [m/s]/1 -> X-Axis Static Friction Model/3(vel [m/s]), X-Axis Kinetic Friction Model/2(vel [m/s])
  X-Axis Kinetic Friction Model/1(posFP [m]) -> X-Axis Static Friction Model/4(posFP [m])
  X-Axis Kinetic Friction Model/3(F_Slide [N]) -> Sum1/2
  X-Axis Static Friction Model/1(F_Stick [N]) -> Sum1/1
  Sum1/1 -> Fx_Friction [N]/1
  Friction Switch/1(Stiction) -> X-Axis Static Friction Model/Enable, Logical Operator/1, Data Type Conversion/1
  X-Axis Static Friction Model/2(Sliding!) -> Friction Switch/1(Slide!)
  X-Axis Kinetic Friction Model/2(Stiction!) -> Friction Switch/2(Stick!)
  Logical Operator/1 -> X-Axis Kinetic Friction Model/Enable
  Data Type Conversion/1 -> Stiction!/1
  Mux1/1 -> Y-Axis Ground Force/1
  Gain3/1 -> Mux1/1
  Gain4/1 -> Mux1/2
  Y-Axis Ground Force/1 -> Fy_Ground[N]/1, X-Axis Static Friction Model/1(F_Normal [N]), X-Axis Kinetic Friction Model/3(F_Normal [N])

== system JenaFox_Klostermair_Neuronal_Controller/Subsystem/knee_l/hard stop extension ==
  note: generate a positive torque to counteract flexion
      | beyond -90°
      | and negative torque to inhibit hyperextension beyond 0°
  phi : Inport
  vphi : Inport  Port=2
  Enable : EnablePort  PropagateVarSize=During execution
  Fcn : Fcn  Expr=c_hs*(0-u[1])-d_hs*u[2]
  Mux : Mux  Inputs=2
  T_hs : Outport  OutputWhenDisabled=reset  InitialOutput=0  VectorParamsAs1DForOutWhenUnconnected=off
  wires:
  phi/1 -> Mux/1
  vphi/1 -> Mux/2
  Mux/1 -> Fcn/1
  Fcn/1 -> T_hs/1

== system JenaFox_Klostermair_Neuronal_Controller/Subsystem/knee_l/hard stop flexion ==
  note: generate a positive torque to counteract flexion
      | beyond -90°
      | and negative torque to inhibit hyperextension beyond 0°
  phi : Inport
  vphi : Inport  Port=2
  Enable : EnablePort  PropagateVarSize=During execution
  Fcn : Fcn  Expr=c_hs*(-92-u[1])-d_hs*u[2]
  Mux : Mux  Inputs=2
  T_hs : Outport  OutputWhenDisabled=reset  InitialOutput=0  VectorParamsAs1DForOutWhenUnconnected=off
  wires:
  Fcn/1 -> T_hs/1
  Mux/1 -> Fcn/1
  vphi/1 -> Mux/2
  phi/1 -> Mux/1

== system JenaFox_Klostermair_Neuronal_Controller/Subsystem/knee_r/hard stop extension ==
  note: generate a positive torque to counteract flexion
      | beyond -90°
      | and negative torque to inhibit hyperextension beyond 0°
  phi : Inport
  vphi : Inport  Port=2
  Enable : EnablePort  PropagateVarSize=During execution
  Fcn : Fcn  Expr=c_hs*(0-u[1])-d_hs*u[2]
  Mux : Mux  Inputs=2
  T_hs : Outport  OutputWhenDisabled=reset  InitialOutput=0  VectorParamsAs1DForOutWhenUnconnected=off
  wires:
  phi/1 -> Mux/1
  vphi/1 -> Mux/2
  Mux/1 -> Fcn/1
  Fcn/1 -> T_hs/1

== system JenaFox_Klostermair_Neuronal_Controller/Subsystem/knee_r/hard stop flexion ==
  note: generate a positive torque to counteract flexion
      | beyond -90°
      | and negative torque to inhibit hyperextension beyond 0°
  phi : Inport
  vphi : Inport  Port=2
  Enable : EnablePort  PropagateVarSize=During execution
  Fcn : Fcn  Expr=c_hs*(-92-u[1])-d_hs*u[2]
  Mux : Mux  Inputs=2
  T_hs : Outport  OutputWhenDisabled=reset  InitialOutput=0  VectorParamsAs1DForOutWhenUnconnected=off
  wires:
  Fcn/1 -> T_hs/1
  Mux/1 -> Fcn/1
  vphi/1 -> Mux/2
  phi/1 -> Mux/1

== system JenaFox_Klostermair_Neuronal_Controller/Subsystem/Ground Contact Model/Ground Friction Model/Friction Switch ==
  note: Static/Kinetic Friction Switch
  Slide! : Inport
  Stick! : Inport  Port=2
  Memory : Memory
  S-R Flip-Flop : simulink_extras/Flip Flops/S-R Flip-Flop  initial_condition=1
  Terminator : Terminator
  Stiction : Outport  VectorParamsAs1DForOutWhenUnconnected=off
  wires:
  S-R Flip-Flop/1 -> Memory/1
  S-R Flip-Flop/2 -> Terminator/1
  Stick!/1 -> S-R Flip-Flop/1
  Slide!/1 -> S-R Flip-Flop/2
  Memory/1 -> Stiction/1

== system JenaFox_Klostermair_Neuronal_Controller/Subsystem/Ground Contact Model/Ground Friction Model/X-Axis Kinetic Friction Model ==
  note: Kinetic Friction Model
  note: Footpoint Determiner
  note: Sliding Limit Detector
  pos [m] : Inport
  vel [m/s] : Inport  Port=2
  F_Normal [N] : Inport  Port=3
  Enable : EnablePort  StatesWhenEnabling=reset  PropagateVarSize=During execution
  Abs : Abs
  Constant : Constant  Value=vLimit
  FixPt Relational Operator : RelationalOperator  Operator=>  OutDataTypeStr=boolean  ZeroCross=off  RndMeth=Nearest
  Memory : Memory  InheritSampleTime=on
  Negative : simulink/Logic and Bit Operations/Compare To Zero  relop=<  OutDataTypeStr=boolean
  Product : Product  RndMeth=Zero
  Sign1 : Signum
  Sum : Sum  Inputs=|+-
  reverse : Gain  Gain=-1
  sliding friction coefficient : Gain  Gain=mu_slide
  posFP [m] : Outport  VectorParamsAs1DForOutWhenUnconnected=off
      settings: AttributesFormatString=initial = '%<InitialOutput>'\nwhen disabled = '%<OutputWhenDisabled>'
  Stiction! : Outport  Port=2  OutputWhenDisabled=reset  InitialOutput=0  VectorParamsAs1DForOutWhenUnconnected=off
      settings: AttributesFormatString=initial = '%<InitialOutput>'\nwhen disabled = '%<OutputWhenDisabled>'
  F_Slide [N] : Outport  Port=3  OutputWhenDisabled=reset  InitialOutput=0  VectorParamsAs1DForOutWhenUnconnected=off
      settings: AttributesFormatString=initial = '%<InitialOutput>'\nwhen disabled = '%<OutputWhenDisabled>'
  wires:
  reverse/1 -> Product/1
  F_Normal [N]/1 -> sliding friction coefficient/1
  vel [m/s]/1 -> Sign1/1, Abs/1
  pos [m]/1 -> posFP [m]/1
  Product/1 -> F_Slide [N]/1
  sliding friction coefficient/1 -> Product/2
  Sign1/1 -> reverse/1
  Memory/1 -> FixPt Relational Operator/2
  Negative/1 -> Memory/1, FixPt Relational Operator/1
  Abs/1 -> Sum/1
  Sum/1 -> Negative/1
  Constant/1 -> Sum/2
  FixPt Relational Operator/1 -> Stiction!/1

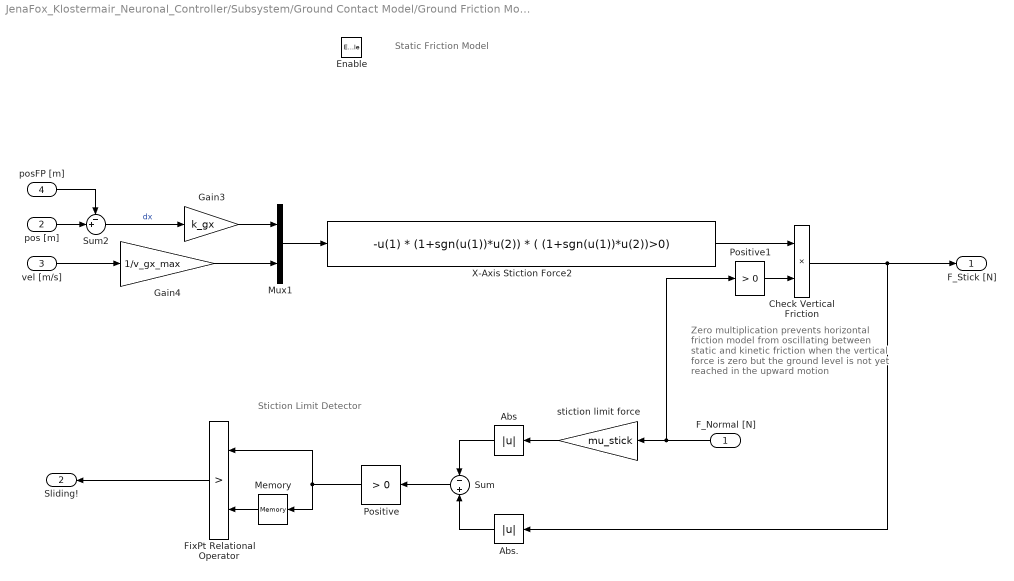
== system JenaFox_Klostermair_Neuronal_Controller/Subsystem/Ground Contact Model/Ground Friction Model/X-Axis Static Friction Model ==
  note: Stiction Limit Detector
  note: Static Friction Model
  note: Zero multiplication prevents
      | horizontal friction model from
      | oscillating between static and kinetic
      | friction when the vertical force is zero but
      | the ground level is not yet reached
      | in the upward motion
  F_Normal [N] : Inport
  pos [m] : Inport  Port=2
  vel [m/s] : Inport  Port=3
  posFP [m] : Inport  Port=4
  Enable : EnablePort  StatesWhenEnabling=reset  PropagateVarSize=During execution
  Abs : Abs
  Abs. : Abs
  Check Vertical Friction : Product  RndMeth=Zero
  FixPt Relational Operator : RelationalOperator  Operator=>  OutDataTypeStr=boolean  ZeroCross=off  RndMeth=Nearest
  Gain3 : Gain  Gain=k_gx
  Gain4 : Gain  Gain=1/v_gx_max
  Memory : Memory
  Mux1 : Mux  Inputs=2
  Positive : simulink/Logic and Bit Operations/Compare To Zero  relop=>  OutDataTypeStr=boolean
  Positive1 : simulink/Logic and Bit Operations/Compare To Zero  relop=>  OutDataTypeStr=boolean
  Sum : Sum  Inputs=-+
  Sum2 : Sum  Inputs=-+|
  X-Axis Stiction Force2 : Fcn  Expr=-u(1) * (1+sgn(u(1))*u(2)) * ( (1+sgn(u(1))*u(2))>0)
  stiction limit force : Gain  Gain=mu_stick
  F_Stick [N] : Outport  OutputWhenDisabled=reset  InitialOutput=0  VectorParamsAs1DForOutWhenUnconnected=off
      settings: AttributesFormatString=when disabled: %<OutputWhenDisabled>\ninitial: %<InitialOutput>
  Sliding! : Outport  Port=2  OutputWhenDisabled=reset  InitialOutput=0  VectorParamsAs1DForOutWhenUnconnected=off
      settings: AttributesFormatString=when disabled: %<OutputWhenDisabled>\ninitial: %<InitialOutput>
  wires:
  F_Normal [N]/1 -> stiction limit force/1, Positive1/1
  Sum2/1 -> Gain3/1  "dx"
  pos [m]/1 -> Sum2/2
  posFP [m]/1 -> Sum2/1
  vel [m/s]/1 -> Gain4/1
  Sum/1 -> Positive/1
  Memory/1 -> FixPt Relational Operator/2
  Positive/1 -> FixPt Relational Operator/1, Memory/1
  Abs./1 -> Sum/2
  Mux1/1 -> X-Axis Stiction Force2/1
  Gain3/1 -> Mux1/1
  Gain4/1 -> Mux1/2
  FixPt Relational Operator/1 -> Sliding!/1
  Abs/1 -> Sum/1
  stiction limit force/1 -> Abs/1
  Positive1/1 -> Check Vertical Friction/2
  Check Vertical Friction/1 -> F_Stick [N]/1, Abs./1
  X-Axis Stiction Force2/1 -> Check Vertical Friction/1

== system JenaFox_Klostermair_Neuronal_Controller/Subsystem/Ground Contact Model1/Ground Friction Model/Friction Switch ==
  note: Static/Kinetic Friction Switch
  Slide! : Inport
  Stick! : Inport  Port=2
  Memory : Memory
  S-R Flip-Flop : simulink_extras/Flip Flops/S-R Flip-Flop  initial_condition=1
  Terminator : Terminator
  Stiction : Outport  VectorParamsAs1DForOutWhenUnconnected=off
  wires:
  S-R Flip-Flop/1 -> Memory/1
  S-R Flip-Flop/2 -> Terminator/1
  Stick!/1 -> S-R Flip-Flop/1
  Slide!/1 -> S-R Flip-Flop/2
  Memory/1 -> Stiction/1

== system JenaFox_Klostermair_Neuronal_Controller/Subsystem/Ground Contact Model1/Ground Friction Model/X-Axis Kinetic Friction Model ==
  note: Kinetic Friction Model
  note: Footpoint Determiner
  note: Sliding Limit Detector
  pos [m] : Inport
  vel [m/s] : Inport  Port=2
  F_Normal [N] : Inport  Port=3
  Enable : EnablePort  StatesWhenEnabling=reset  PropagateVarSize=During execution
  Abs : Abs
  Constant : Constant  Value=vLimit
  FixPt Relational Operator : RelationalOperator  Operator=>  OutDataTypeStr=boolean  ZeroCross=off  RndMeth=Nearest
  Memory : Memory  InheritSampleTime=on
  Negative : simulink/Logic and Bit Operations/Compare To Zero  relop=<  OutDataTypeStr=boolean
  Product : Product  RndMeth=Zero
  Sign1 : Signum
  Sum : Sum  Inputs=|+-
  reverse : Gain  Gain=-1
  sliding friction coefficient : Gain  Gain=mu_slide
  posFP [m] : Outport  VectorParamsAs1DForOutWhenUnconnected=off
      settings: AttributesFormatString=initial = '%<InitialOutput>'\nwhen disabled = '%<OutputWhenDisabled>'
  Stiction! : Outport  Port=2  OutputWhenDisabled=reset  InitialOutput=0  VectorParamsAs1DForOutWhenUnconnected=off
      settings: AttributesFormatString=initial = '%<InitialOutput>'\nwhen disabled = '%<OutputWhenDisabled>'
  F_Slide [N] : Outport  Port=3  OutputWhenDisabled=reset  InitialOutput=0  VectorParamsAs1DForOutWhenUnconnected=off
      settings: AttributesFormatString=initial = '%<InitialOutput>'\nwhen disabled = '%<OutputWhenDisabled>'
  wires:
  reverse/1 -> Product/1
  F_Normal [N]/1 -> sliding friction coefficient/1
  vel [m/s]/1 -> Sign1/1, Abs/1
  pos [m]/1 -> posFP [m]/1
  Product/1 -> F_Slide [N]/1
  sliding friction coefficient/1 -> Product/2
  Sign1/1 -> reverse/1
  Memory/1 -> FixPt Relational Operator/2
  Negative/1 -> Memory/1, FixPt Relational Operator/1
  Abs/1 -> Sum/1
  Sum/1 -> Negative/1
  Constant/1 -> Sum/2
  FixPt Relational Operator/1 -> Stiction!/1

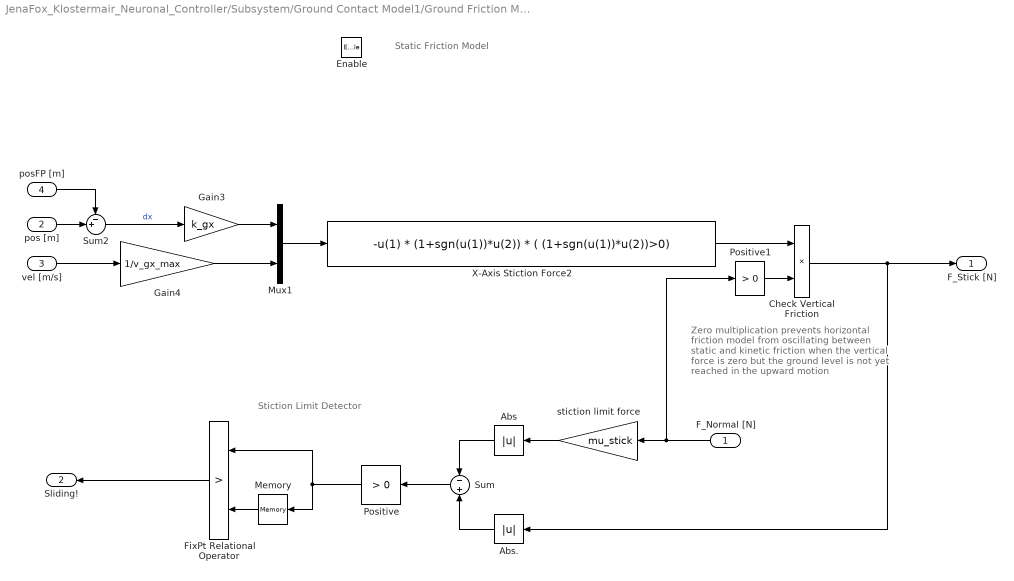
== system JenaFox_Klostermair_Neuronal_Controller/Subsystem/Ground Contact Model1/Ground Friction Model/X-Axis Static Friction Model ==
  note: Stiction Limit Detector
  note: Static Friction Model
  note: Zero multiplication prevents
      | horizontal friction model from
      | oscillating between static and kinetic
      | friction when the vertical force is zero but
      | the ground level is not yet reached
      | in the upward motion
  F_Normal [N] : Inport
  pos [m] : Inport  Port=2
  vel [m/s] : Inport  Port=3
  posFP [m] : Inport  Port=4
  Enable : EnablePort  StatesWhenEnabling=reset  PropagateVarSize=During execution
  Abs : Abs
  Abs. : Abs
  Check Vertical Friction : Product  RndMeth=Zero
  FixPt Relational Operator : RelationalOperator  Operator=>  OutDataTypeStr=boolean  ZeroCross=off  RndMeth=Nearest
  Gain3 : Gain  Gain=k_gx
  Gain4 : Gain  Gain=1/v_gx_max
  Memory : Memory
  Mux1 : Mux  Inputs=2
  Positive : simulink/Logic and Bit Operations/Compare To Zero  relop=>  OutDataTypeStr=boolean
  Positive1 : simulink/Logic and Bit Operations/Compare To Zero  relop=>  OutDataTypeStr=boolean
  Sum : Sum  Inputs=-+
  Sum2 : Sum  Inputs=-+|
  X-Axis Stiction Force2 : Fcn  Expr=-u(1) * (1+sgn(u(1))*u(2)) * ( (1+sgn(u(1))*u(2))>0)
  stiction limit force : Gain  Gain=mu_stick
  F_Stick [N] : Outport  OutputWhenDisabled=reset  InitialOutput=0  VectorParamsAs1DForOutWhenUnconnected=off
      settings: AttributesFormatString=when disabled: %<OutputWhenDisabled>\ninitial: %<InitialOutput>
  Sliding! : Outport  Port=2  OutputWhenDisabled=reset  InitialOutput=0  VectorParamsAs1DForOutWhenUnconnected=off
      settings: AttributesFormatString=when disabled: %<OutputWhenDisabled>\ninitial: %<InitialOutput>
  wires:
  F_Normal [N]/1 -> stiction limit force/1, Positive1/1
  Sum2/1 -> Gain3/1  "dx"
  pos [m]/1 -> Sum2/2
  posFP [m]/1 -> Sum2/1
  vel [m/s]/1 -> Gain4/1
  Sum/1 -> Positive/1
  Memory/1 -> FixPt Relational Operator/2
  Positive/1 -> FixPt Relational Operator/1, Memory/1
  Abs./1 -> Sum/2
  Mux1/1 -> X-Axis Stiction Force2/1
  Gain3/1 -> Mux1/1
  Gain4/1 -> Mux1/2
  FixPt Relational Operator/1 -> Sliding!/1
  Abs/1 -> Sum/1
  stiction limit force/1 -> Abs/1
  Positive1/1 -> Check Vertical Friction/2
  Check Vertical Friction/1 -> F_Stick [N]/1, Abs./1
  X-Axis Stiction Force2/1 -> Check Vertical Friction/1
